simulink model "EvBoltCalib_Lat_v1_comb_GBS"  (R2022b)
settings: configuration reference "ConfigSetDesktopFixedStep" (kept outside this file)
PreLoadFcn:
  | VSS_BICYCLE=Simulink.Variant('Dual=0');
  | VSS_DUAL=Simulink.Variant('Dual=1');
  | Dual=1;
model workspace (MAT data in the model file):
  Gas = 0.383333333333
undefined symbols (not defined in the file or in its folder): AccelCmd, BattChargeLimitMaxPwr, BattChargeLimitSocBpts, BattChargeLimitTbl, BattChrgCapcty, BattDischargeLimitSocBpts, BattDischargeLimitTbl, BattDischargeMaxPwr, BattNumCellsParallel, BattNumCellsSeries, BattOpenVoltCapBpts, BattOpenVoltTbl, BattResistSocBpts, BattResistTbl, BattResistTempBpts, BrakeMaxPrs, BrakeMaxTrq, ChassisDistCg2FrontAxle, ChassisDistCg2RearAxle, ChassisVehMass, CltchCmd, DecelCmd, DiffRatio, EnvGravCnst, EnvPrs, EnvTemp, FuelSpecificGrav, GearCmd, h, InitStates, lgSw, MtrEffSpdBpts, MtrEffTbl, MtrEffTrqBpts, MtrPwrMax, MtrTrqMax, SteeringCmd, SupvsryCtrlRegenBrkCutOffTbl, SupvsryCtrlRegenSpdBpts, TestScnrioCycleNum, VEH
libraries: vehdynlibtire x8, vehdynlibsuspension x7, simulink x6, autolibutils x5, autolibshared x5, VsrLibWheel x4, vehdynlibtirecommon x3, sharedtransform x3, slrealtimeiplib x3, slrealtimeutilitieslib x2, autolibbatterycommon x2, autolibpowerinfoutils x2
(part 7 of 9)

== system EvBoltCalib_Lat_v1_comb_GBS/Subsystem/Vehicle/Vehicle Dynamics/Vehicle 7DOF/Longitudinal Wheels 4DOF/Velocity and Vertical Load/Dual ==
  VehFdbk : Inport
  Dual Fz : Subsystem
  Dual V : Subsystem
  VehVel : Outport  VectorParamsAs1DForOutWhenUnconnected=off
  Fz : Outport  Port=2  VectorParamsAs1DForOutWhenUnconnected=off
  wires:
  Dual V/1(Out1) -> VehVel/1
  VehFdbk/1 -> Dual Fz/1(In1), Dual V/1(In1)
  Dual Fz/1(Out1) -> Fz/1

== system EvBoltCalib_Lat_v1_comb_GBS/Subsystem/Vehicle/Vehicle Dynamics/Vehicle 7DOF/Vehicle Body 3DOF External Longitudinal Wheels/Bicycle/Wheel Positions ==
  Info : Inport
  Bus Selector : BusSelector  OutputSignals=InertFrm.FrntAxl.Disp.Y,InertFrm.RearAxl.Disp.Y
  Bus Selector1 : BusSelector  OutputSignals=InertFrm.FrntAxl.Disp.X,InertFrm.RearAxl.Disp.X
  Constant : Constant  Value=0
  Constant1 : Constant  Value=0
  Vector Concatenate1 : Concatenate  NumInputs=4
  Vector Concatenate2 : Concatenate  NumInputs=4
  XWheel : Outport  Unit=m  VectorParamsAs1DForOutWhenUnconnected=off
  YWheel : Outport  Port=2  Unit=m  VectorParamsAs1DForOutWhenUnconnected=off
  wires:
  Constant1/1 -> Vector Concatenate1/4, Vector Concatenate1/2
  Vector Concatenate1/1 -> YWheel/1
  Bus Selector/2 -> Vector Concatenate1/3  "<Y>"
  Bus Selector/1 -> Vector Concatenate1/1  "<Y>"
  Constant/1 -> Vector Concatenate2/4, Vector Concatenate2/2
  Info/1 -> Bus Selector/1, Bus Selector1/1
  Vector Concatenate2/1 -> XWheel/1
  Bus Selector1/2 -> Vector Concatenate2/3  "<X>"
  Bus Selector1/1 -> Vector Concatenate2/1  "<X>"

== system EvBoltCalib_Lat_v1_comb_GBS/Subsystem/Vehicle/Vehicle Dynamics/Vehicle 7DOF/Vehicle Body 3DOF External Longitudinal Wheels/Dual/Wheel Positions ==
  Info : Inport
  Bus Selector : BusSelector  OutputSignals=InertFrm.FrntAxl.Lft.Disp.Y,InertFrm.FrntAxl.Rght.Disp.Y,InertFrm.RearAxl.Lft.Disp.Y,InertFrm.RearAxl.Rght.Disp.Y
  Bus Selector1 : BusSelector  OutputSignals=InertFrm.FrntAxl.Lft.Disp.X,InertFrm.FrntAxl.Rght.Disp.X,InertFrm.RearAxl.Lft.Disp.X,InertFrm.RearAxl.Rght.Disp.X
  Vector Concatenate1 : Concatenate  NumInputs=4
  Vector Concatenate2 : Concatenate  NumInputs=4
  XWheel : Outport  Unit=m  VectorParamsAs1DForOutWhenUnconnected=off
  YWheel : Outport  Port=2  Unit=m  VectorParamsAs1DForOutWhenUnconnected=off
  wires:
  Bus Selector1/4 -> Vector Concatenate2/4  "<X>"
  Bus Selector/1 -> Vector Concatenate1/1  "<Y>"
  Bus Selector1/3 -> Vector Concatenate2/3  "<X>"
  Bus Selector/4 -> Vector Concatenate1/4  "<Y>"
  Bus Selector1/2 -> Vector Concatenate2/2  "<X>"
  Bus Selector/3 -> Vector Concatenate1/3  "<Y>"
  Bus Selector/2 -> Vector Concatenate1/2  "<Y>"
  Vector Concatenate1/1 -> YWheel/1
  Info/1 -> Bus Selector/1, Bus Selector1/1
  Bus Selector1/1 -> Vector Concatenate2/1  "<X>"
  Vector Concatenate2/1 -> XWheel/1

== system EvBoltCalib_Lat_v1_comb_GBS/Subsystem/Vehicle/Battery/Battery/Lithium Ion Battery Pack1/Datasheet Battery Internal/Datasheet Battery/Charge Model ==
  LdAmp : Inport
  CapInit : Inport  Port=2
  Constant1 : Constant  Value=BattChargeMax
  Gain1 : Gain  Gain=-1/(Np*3600)
  Integrator Limited : Integrator  InitialConditionSource=external  InitialCondition=BattCapInit  LimitOutput=on  UpperSaturationLimit=BattChargeMax  LowerSaturationLimit=0
  Switch : Switch  Criteria=u2 > Threshold  Threshold=BattChargeMax  SaturateOnIntegerOverflow=off  InputSameDT=off
  LdAmpHr : Outport  VectorParamsAs1DForOutWhenUnconnected=off
  wires:
  Switch/1 -> Integrator Limited/2
  Constant1/1 -> Switch/1
  CapInit/1 -> Switch/2, Switch/3
  LdAmp/1 -> Gain1/1
  Integrator Limited/1 -> LdAmpHr/1
  Gain1/1 -> Integrator Limited/1

== system EvBoltCalib_Lat_v1_comb_GBS/Subsystem/Vehicle/Battery/Battery/Lithium Ion Battery Pack1/Datasheet Battery Internal/Datasheet Battery/State of Charge Capacity ==
  LdAmpHr : Inport
  Constant1 : Constant  Value=BattChargeMax
  Divide : Product  Inputs=*/
  CapSOC : Outport  VectorParamsAs1DForOutWhenUnconnected=off
  wires:
  Divide/1 -> CapSOC/1
  LdAmpHr/1 -> Divide/1
  Constant1/1 -> Divide/2

== system EvBoltCalib_Lat_v1_comb_GBS/Subsystem/Vehicle/Battery/Battery/Lithium Ion Battery Pack1/Datasheet Battery Internal/Datasheet Battery/Voltage and Power Calculation ==
  CapSOC : Inport
  LdAmp : Inport  Port=2
  BattTemp : Inport  Port=3
  Em : Lookup_n-D  NumberOfTableDimensions=1  LookupTableObject=''  BreakpointsForDimension1=CapLUTBp  BreakpointsForDimension2=CapSOCBp  Table=Em  ExtrapMethod=Clip  UseLastTableValue=on  InternalRulePriority=Speed  RndMeth=Simplest
  Gain1 : Gain  Gain=Ns
  Gain2 : Gain  Gain=1/Np
  Gain3 : Gain  Gain=Ns
  Gain4 : Gain  Gain=Np
  Product : Product
  Product1 : Product
  R : Lookup_n-D  LookupTableObject=''  BreakpointsForDimension1=BattTempBp  BreakpointsForDimension2=CapSOCBp  Table=RInt  ExtrapMethod=Clip  UseLastTableValue=on  InternalRulePriority=Speed  RndMeth=Simplest
      settings: InputPortMap=u0,u1
  Subtract : Sum  Inputs=+-
  OutVolt : Outport  VectorParamsAs1DForOutWhenUnconnected=off
  BattPwrLoss : Outport  Port=2  VectorParamsAs1DForOutWhenUnconnected=off
  wires:
  Gain4/1 -> BattPwrLoss/1
  Gain3/1 -> Gain4/1
  Product1/1 -> Gain3/1
  Gain2/1 -> Product/2, Product1/2
  CapSOC/1 -> R/2, Em/1
  LdAmp/1 -> Gain2/1
  Subtract/1 -> Gain1/1
  BattTemp/1 -> R/1
  Product/1 -> Subtract/2, Product1/1
  R/1 -> Product/1
  Em/1 -> Subtract/1
  Gain1/1 -> OutVolt/1

== system EvBoltCalib_Lat_v1_comb_GBS/Subsystem/Vehicle/Vehicle Dynamics/Vehicle 14DOF/Wheels and Tires/VDBS/Tire2Veh/Routiong ==
  <Mz> : Inport
  <Mx> : Inport  Port=2
  <My> : Inport  Port=3
  <Re> : Inport  Port=4
  <z> : Inport  Port=5
  <zdot> : Inport  Port=6
  <Kappa> : Inport  Port=7
  <Alpha> : Inport  Port=8
  Omega : Inport  Port=9
  Fx : Inport  Port=10
  Fy : Inport  Port=11
  Fz : Inport  Port=12
  Bus Creator : BusCreator  Inputs=12
  Reshape : Reshape  OutputDimensionality=Row vector (2-D)
  Reshape1 : Reshape  OutputDimensionality=Row vector (2-D)
  Unary Minus1 : UnaryMinus
  Unary Minus2 : UnaryMinus
  Out1 : Outport  VectorParamsAs1DForOutWhenUnconnected=off
  Out2 : Outport  Port=2  VectorParamsAs1DForOutWhenUnconnected=off
  Out3 : Outport  Port=3  VectorParamsAs1DForOutWhenUnconnected=off
  wires:
  <Re>/1 -> Bus Creator/8
  Unary Minus1/1 -> Reshape/1, Bus Creator/9  "z"
  Fz/1 -> Bus Creator/4
  <zdot>/1 -> Unary Minus2/1
  <Mz>/1 -> Bus Creator/7
  Unary Minus2/1 -> Reshape1/1, Bus Creator/10  "zdot"
  <z>/1 -> Unary Minus1/1
  Bus Creator/1 -> Out1/1
  Fy/1 -> Bus Creator/3
  Omega/1 -> Bus Creator/1  "Omega"
  Fx/1 -> Bus Creator/2
  Reshape1/1 -> Out3/1
  <Kappa>/1 -> Bus Creator/11
  Reshape/1 -> Out2/1
  <Mx>/1 -> Bus Creator/5
  <My>/1 -> Bus Creator/6
  <Alpha>/1 -> Bus Creator/12

== system EvBoltCalib_Lat_v1_comb_GBS/Subsystem/Vehicle/Vehicle Dynamics/Vehicle 14DOF/Wheels and Tires/VDBS/Tire2Veh/Wheel Angles ==
  Front : Inport
  Camber : Inport  Port=2
  Add1 : Sum
  Add2 : Sum
  Constant1 : Constant  Value=pi
  Constant2 : Constant  Value=[pi;0;pi;0].*0+[0;pi;0;pi].*.0
  Constant3 : Constant  Value=ones(1,4).*0
  Reshape : Reshape  OutputDimensionality=Row vector (2-D)
  Reshape1 : Reshape  OutputDimensionality=Row vector (2-D)
  Reshape2 : Reshape  OutputDimensionality=Row vector (2-D)
  Vector Concatenate3 : Concatenate  NumInputs=3  Mode=Multidimensional array
  Vehicle : Outport  VectorParamsAs1DForOutWhenUnconnected=off
  wires:
  Reshape/1 -> Vector Concatenate3/3
  Reshape2/1 -> Vector Concatenate3/2
  Vector Concatenate3/1 -> Vehicle/1
  Constant2/1 -> Add1/2
  Front/1 -> Add1/1
  Reshape1/1 -> Vector Concatenate3/1
  Constant3/1 -> Reshape2/1
  Add1/1 -> Reshape/1
  Camber/1 -> Add2/1
  Add2/1 -> Reshape1/1
  Constant1/1 -> Add2/2

== system EvBoltCalib_Lat_v1_comb_GBS/Subsystem/Vehicle/Vehicle Dynamics/Vehicle 14DOF/Wheels and Tires/VDBS/Tire2Veh/Wheel to Body Transform ==
  Forces : Inport  Partition=on  PartitionDimension=2  PartitionWidth=1  PartitionOffset=0
  WheelAngles : Inport  Port=2  Partition=on  PartitionDimension=2  PartitionWidth=1  PartitionOffset=0
  Demux1 : Demux  Outputs=3
  Divide1 : Product  Inputs=**  Multiplication=Matrix(*)
  For Each : ForEach  DisableCoverage=on
  Rotation Angles to Direction Cosine Matrix : sharedtransform/Rotation Angles to Direction Cosine Matrix  rotationOrder=ZYX  aMode=2
  Selector : Selector  InputPortWidth=3  IndexOptions=Index vector (dialog)  Indices=[3 2 1]  OutputSizes=1
  Fx : Outport  ConcatenationDimension=1  VectorParamsAs1DForOutWhenUnconnected=off
  Fy : Outport  Port=2  ConcatenationDimension=1  VectorParamsAs1DForOutWhenUnconnected=off
  Fz : Outport  Port=3  ConcatenationDimension=1  VectorParamsAs1DForOutWhenUnconnected=off
  wires:
  Divide1/1 -> Demux1/1
  Demux1/1 -> Fx/1
  Demux1/2 -> Fy/1
  Demux1/3 -> Fz/1
  Rotation Angles to Direction Cosine Matrix/1 -> Divide1/1
  Forces/1 -> Divide1/2
  WheelAngles/1 -> Selector/1
  Selector/1 -> Rotation Angles to Direction Cosine Matrix/1
